simulink model "robot_TR4_joint"  (R2020a)
settings: Solver=ode15s  StartTime=0.0  StopTime=20.1113  RelTol=1e-3
undefined symbols (not defined in the file): dT_target, Fq_interp, Q_interp, Qp_interp, Qpp_interp, X, Y, Z
libraries: nesl_utility x25, sm_lib x18
settings Model: Creator=monti  LastModifiedBy=campr
settings DebuggingCC: SFMachineParentedDataDiag=error

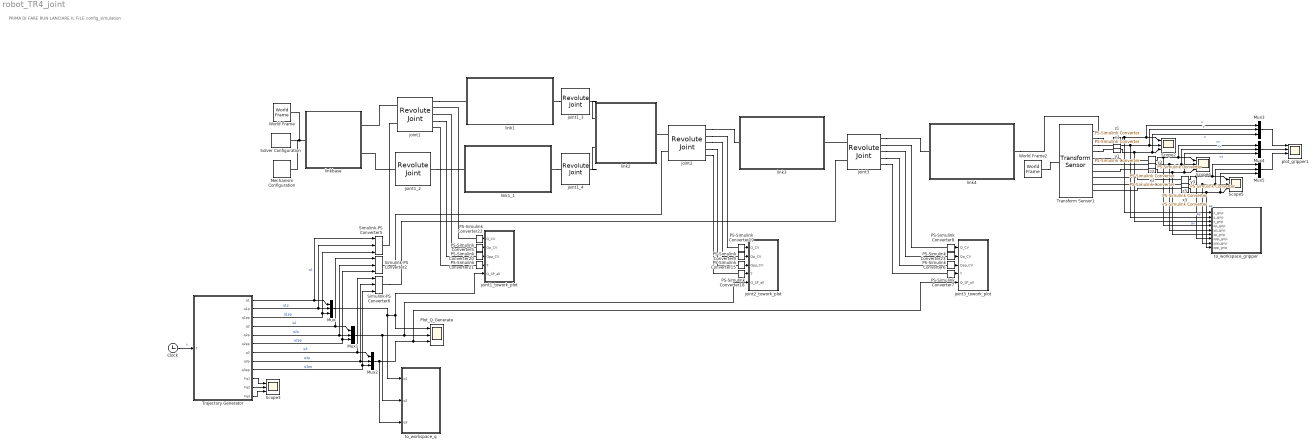
== system robot_TR4_joint ==
  note: PRIMA DI FARE RUN LANCIARE IL FILE config_simulation
  Clock : Clock
  Mechanism Configuration : sm_lib/Utilities/Mechanism Configuration  UniformGravity=Constant  GravityVector=[0 -9.80665 0]  GravityVectorUnits=m/s^2  GravityUnits=m/s^2  LinearizationDelta=0.001  JointModeTransitionNonlinearIterations=2
  Mux{,1..5} (6 alike) : Mux  Inputs=3
  PS-Simulink Converter15 : nesl_utility/PS-Simulink Converter  PhysicalDomain=network_engine_domain  SubClassName=ps_output  LeftPortType=input  RightPortType=output  PseudoPeriodic=off  Frequencies=[]  Unit=rad/s^2  AffineConversion=off
  PS-Simulink Converter18 : nesl_utility/PS-Simulink Converter  PhysicalDomain=network_engine_domain  SubClassName=ps_output  LeftPortType=input  RightPortType=output  PseudoPeriodic=off  Frequencies=[]  Unit=N*m  AffineConversion=off
  PS-Simulink Converter19 : nesl_utility/PS-Simulink Converter  PhysicalDomain=network_engine_domain  SubClassName=ps_output  LeftPortType=input  RightPortType=output  PseudoPeriodic=off  Frequencies=[]  Unit=rad  AffineConversion=off
  PS-Simulink Converter20 : nesl_utility/PS-Simulink Converter  PhysicalDomain=network_engine_domain  SubClassName=ps_output  LeftPortType=input  RightPortType=output  PseudoPeriodic=off  Frequencies=[]  Unit=rad/s^2  AffineConversion=off
  PS-Simulink Converter21 : nesl_utility/PS-Simulink Converter  PhysicalDomain=network_engine_domain  SubClassName=ps_output  LeftPortType=input  RightPortType=output  PseudoPeriodic=off  Frequencies=[]  Unit=N*m  AffineConversion=off
  PS-Simulink Converter22 : nesl_utility/PS-Simulink Converter  PhysicalDomain=network_engine_domain  SubClassName=ps_output  LeftPortType=input  RightPortType=output  PseudoPeriodic=off  Frequencies=[]  Unit=rad  AffineConversion=off
  PS-Simulink Converter23 : nesl_utility/PS-Simulink Converter  PhysicalDomain=network_engine_domain  SubClassName=ps_output  LeftPortType=input  RightPortType=output  PseudoPeriodic=off  Frequencies=[]  Unit=rad/s  AffineConversion=off
  PS-Simulink Converter5 : nesl_utility/PS-Simulink Converter  PhysicalDomain=network_engine_domain  SubClassName=ps_output  LeftPortType=input  RightPortType=output  PseudoPeriodic=off  Frequencies=[]  Unit=rad/s  AffineConversion=off
  PS-Simulink Converter6 : nesl_utility/PS-Simulink Converter  PhysicalDomain=network_engine_domain  SubClassName=ps_output  LeftPortType=input  RightPortType=output  PseudoPeriodic=off  Frequencies=[]  Unit=rad/s^2  AffineConversion=off
  PS-Simulink Converter7 : nesl_utility/PS-Simulink Converter  PhysicalDomain=network_engine_domain  SubClassName=ps_output  LeftPortType=input  RightPortType=output  PseudoPeriodic=off  Frequencies=[]  Unit=N*m  AffineConversion=off
  PS-Simulink Converter8 : nesl_utility/PS-Simulink Converter  PhysicalDomain=network_engine_domain  SubClassName=ps_output  LeftPortType=input  RightPortType=output  PseudoPeriodic=off  Frequencies=[]  Unit=rad  AffineConversion=off
  PS-Simulink Converter9 : nesl_utility/PS-Simulink Converter  PhysicalDomain=network_engine_domain  SubClassName=ps_output  LeftPortType=input  RightPortType=output  PseudoPeriodic=off  Frequencies=[]  Unit=rad/s  AffineConversion=off
  Plot_Q_Generate : Scope  NumInputPorts=3
  Scope{2..5} (4 alike) : Scope  NumInputPorts=3
  Simulink-PS Converter2 : nesl_utility/Simulink-PS Converter  PhysicalDomain=network_engine_domain  SubClassName=ps_input  LeftPortType=input  RightPortType=output  PseudoPeriodic=off  Frequencies=[]  NoiseDistribution=none  NoiseParameters=[]  Unit=rad  AffineConversion=off  FilteringAndDerivatives=provide  SimscapeFilterOrder=1  InputFilterTimeConstant=0.001  UdotUserProvided=2
  Simulink-PS Converter5 : nesl_utility/Simulink-PS Converter  PhysicalDomain=network_engine_domain  SubClassName=ps_input  LeftPortType=input  RightPortType=output  PseudoPeriodic=off  Frequencies=[]  NoiseDistribution=none  NoiseParameters=[]  Unit=rad  AffineConversion=off  FilteringAndDerivatives=provide  SimscapeFilterOrder=1  InputFilterTimeConstant=0.001  UdotUserProvided=2
  Simulink-PS Converter6 : nesl_utility/Simulink-PS Converter  PhysicalDomain=network_engine_domain  SubClassName=ps_input  LeftPortType=input  RightPortType=output  PseudoPeriodic=off  Frequencies=[]  NoiseDistribution=none  NoiseParameters=[]  Unit=rad  AffineConversion=off  FilteringAndDerivatives=provide  SimscapeFilterOrder=1  InputFilterTimeConstant=0.001  UdotUserProvided=2
  Solver Configuration : nesl_utility/Solver Configuration  PhysicalDomain=network_engine_domain  SubClassName=solver  LeftPortType=input  RightPortType=generic  Tones=[]  Harmonics=[]  SimulateNoise=off  Profile=off  UseLocalSampling=off  EnableSwitchedLinearOptims=on  FrequencyDomain=off  UseCCode=off  RelTol=0.001  AbsTol=1e-06  MinStep=1e-09  ToWorkspace=off  RevertToSquareIcSolve=off  NumHomotopyIterations=100  PhasorMode=off  PhasorModeNumHarmonics=1  DoDC=off  ResidualTolerance=1e-5  UseLocalSolver=off  LocalSolverChoice=NE_BACKWARD_EULER_ADVANCER  LocalSolverSampleTime=0.001  DoFixedCost=off  MaxNonlinIter=3  MaxModeIter=2  ComputeImpulses=off  ImpulseIterations=2  LinearAlgebra=Sparse  EquationFormulation=NE_TIME_EF  DelaysMemoryBudget=1024  AutomaticFiltering=on  FilteringTimeConstant=0.001  PartitionStorageMethod=AS_NEEDED  PartitionMemoryBudget=1024  PartitionMethod=FAST
  Trajectory Generator : MATLAB Function  TreatAsAtomicUnit=on
  Transform Sensor1 : sm_lib/Frames and Transforms/Transform Sensor  MeasurementFrame=World  SenseAngle=off  SenseAxis=off  SenseAngle1=off  SenseAngle2=off  SenseAngle3=off  SenseQ=off  SenseR=off  SenseOmegaX=off  SenseOmegaY=off  SenseOmegaZ=off  SenseOmega1=off  SenseOmega2=off  SenseOmega3=off  SenseQDot=off  SenseRDot=off  SenseAlphaX=off  SenseAlphaY=off  SenseAlphaZ=off  SenseAlpha1=off  SenseAlpha2=off  SenseAlpha3=off  SenseQDDot=off  SenseRDDot=off  SenseX=on  SenseY=on  SenseZ=on  SenseRad=off  SenseAzim=off  SenseDist=off  SenseInc=off  SenseXDot=on  SenseYDot=on  SenseZDot=on  SenseRadDot=off  SenseAzimDot=off  SenseDistDot=off  SenseIncDot=off  SenseXDDot=on  SenseYDDot=on  SenseZDDot=on  SenseRadDDot=off  SenseAzimDDot=off  SenseDistDDot=off  SenseIncDDot=off
  World Frame : sm_lib/Frames and Transforms/World Frame
  World Frame2 : sm_lib/Frames and Transforms/World Frame
  joint1 : sm_lib/Joints/Revolute Joint  JointMode=Normal  SenseConstraintForce=off  SenseConstraintForceX=off  SenseConstraintForceY=off  SenseConstraintForceZ=off  SenseConstraintTorque=off  SenseConstraintTorqueX=off  SenseConstraintTorqueY=off  SenseConstraintTorqueZ=off  SenseTotalForce=off  SenseTotalForceX=off  SenseTotalForceY=off  SenseTotalForceZ=off  SenseTotalTorque=off  SenseTotalTorqueX=off  SenseTotalTorqueY=off  SenseTotalTorqueZ=off  CompositeWrenchDir=FollowerOnBase  CompositeWrenchFrame=BaseFrame  EquilibriumPosition=0  EquilibriumPositionUnits=rad  SpringStiffness=0  SpringStiffnessUnits=N*m/deg  DampingCoefficient=0  DampingCoefficientUnits=N*m/(deg/s)  TorqueActuationMode=ComputedTorque  MotionActuationMode=InputMotion  SensePosition=on  SenseVelocity=on  SenseAcceleration=on  SenseTorqueForce=on  SenseLowerLimitTorqueForce=off  SenseUpperLimitTorqueForce=off  LowerLimitSpecify=on  LowerLimitBound=-1.5708  LowerLimitBoundUnits=rad  LowerLimitStiffness=0  LowerLimitStiffnessUnits=N*m/deg  LowerLimitDamping=0  LowerLimitDampingUnits=N*m/(deg/s)  LowerLimitTransitionRegionWidth=0.1  LowerLimitTransitionRegionWidthUnits=deg  UpperLimitSpecify=on  UpperLimitBound=1.5708  UpperLimitBoundUnits=rad  UpperLimitStiffness=0  UpperLimitStiffnessUnits=N*m/deg  UpperLimitDamping=0  UpperLimitDampingUnits=N*m/(deg/s)  UpperLimitTransitionRegionWidth=0.1  UpperLimitTransitionRegionWidthUnits=deg  PositionTargetSpecify=on  PositionTargetPriority=High  PositionTargetValue=0.5236  PositionTargetValueUnits=rad  VelocityTargetSpecify=off  VelocityTargetPriority=High  VelocityTargetValue=10  VelocityTargetValueUnits=deg/s
  joint1_2 : sm_lib/Joints/Revolute Joint  JointMode=Normal  SenseConstraintForce=off  SenseConstraintForceX=off  SenseConstraintForceY=off  SenseConstraintForceZ=off  SenseConstraintTorque=off  SenseConstraintTorqueX=off  SenseConstraintTorqueY=off  SenseConstraintTorqueZ=off  SenseTotalForce=off  SenseTotalForceX=off  SenseTotalForceY=off  SenseTotalForceZ=off  SenseTotalTorque=off  SenseTotalTorqueX=off  SenseTotalTorqueY=off  SenseTotalTorqueZ=off  CompositeWrenchDir=FollowerOnBase  CompositeWrenchFrame=BaseFrame  EquilibriumPosition=0  EquilibriumPositionUnits=deg  SpringStiffness=0  SpringStiffnessUnits=N*m/deg  DampingCoefficient=0  DampingCoefficientUnits=N*m/(deg/s)  TorqueActuationMode=NoTorque  MotionActuationMode=ComputedMotion  SensePosition=off  SenseVelocity=off  SenseAcceleration=off  SenseTorqueForce=off  SenseLowerLimitTorqueForce=off  SenseUpperLimitTorqueForce=off  LowerLimitSpecify=off  LowerLimitBound=-1.5708  LowerLimitBoundUnits=rad  LowerLimitStiffness=1e4  LowerLimitStiffnessUnits=N*m/deg  LowerLimitDamping=10  LowerLimitDampingUnits=N*m/(deg/s)  LowerLimitTransitionRegionWidth=0.1  LowerLimitTransitionRegionWidthUnits=deg  UpperLimitSpecify=off  UpperLimitBound=1.5708  UpperLimitBoundUnits=rad  UpperLimitStiffness=1e4  UpperLimitStiffnessUnits=N*m/deg  UpperLimitDamping=10  UpperLimitDampingUnits=N*m/(deg/s)  UpperLimitTransitionRegionWidth=0.1  UpperLimitTransitionRegionWidthUnits=deg  PositionTargetSpecify=on  PositionTargetPriority=High  PositionTargetValue=0.5236  PositionTargetValueUnits=rad  VelocityTargetSpecify=off  VelocityTargetPriority=High  VelocityTargetValue=0  VelocityTargetValueUnits=deg/s
  joint1_3 : sm_lib/Joints/Revolute Joint  JointMode=Normal  SenseConstraintForce=off  SenseConstraintForceX=off  SenseConstraintForceY=off  SenseConstraintForceZ=off  SenseConstraintTorque=off  SenseConstraintTorqueX=off  SenseConstraintTorqueY=off  SenseConstraintTorqueZ=off  SenseTotalForce=off  SenseTotalForceX=off  SenseTotalForceY=off  SenseTotalForceZ=off  SenseTotalTorque=off  SenseTotalTorqueX=off  SenseTotalTorqueY=off  SenseTotalTorqueZ=off  CompositeWrenchDir=FollowerOnBase  CompositeWrenchFrame=BaseFrame  EquilibriumPosition=0  EquilibriumPositionUnits=deg  SpringStiffness=0  SpringStiffnessUnits=N*m/deg  DampingCoefficient=0  DampingCoefficientUnits=N*m/(deg/s)  TorqueActuationMode=NoTorque  MotionActuationMode=ComputedMotion  SensePosition=off  SenseVelocity=off  SenseAcceleration=off  SenseTorqueForce=off  SenseLowerLimitTorqueForce=off  SenseUpperLimitTorqueForce=off  LowerLimitSpecify=off  LowerLimitBound=-90  LowerLimitBoundUnits=deg  LowerLimitStiffness=1e4  LowerLimitStiffnessUnits=N*m/deg  LowerLimitDamping=10  LowerLimitDampingUnits=N*m/(deg/s)  LowerLimitTransitionRegionWidth=0.1  LowerLimitTransitionRegionWidthUnits=deg  UpperLimitSpecify=off  UpperLimitBound=90  UpperLimitBoundUnits=deg  UpperLimitStiffness=1e4  UpperLimitStiffnessUnits=N*m/deg  UpperLimitDamping=10  UpperLimitDampingUnits=N*m/(deg/s)  UpperLimitTransitionRegionWidth=0.1  UpperLimitTransitionRegionWidthUnits=deg  PositionTargetSpecify=off  PositionTargetPriority=High  PositionTargetValue=0  PositionTargetValueUnits=deg  VelocityTargetSpecify=off  VelocityTargetPriority=High  VelocityTargetValue=0  VelocityTargetValueUnits=deg/s
  joint1_4 : sm_lib/Joints/Revolute Joint  JointMode=Normal  SenseConstraintForce=off  SenseConstraintForceX=off  SenseConstraintForceY=off  SenseConstraintForceZ=off  SenseConstraintTorque=off  SenseConstraintTorqueX=off  SenseConstraintTorqueY=off  SenseConstraintTorqueZ=off  SenseTotalForce=off  SenseTotalForceX=off  SenseTotalForceY=off  SenseTotalForceZ=off  SenseTotalTorque=off  SenseTotalTorqueX=off  SenseTotalTorqueY=off  SenseTotalTorqueZ=off  CompositeWrenchDir=FollowerOnBase  CompositeWrenchFrame=BaseFrame  EquilibriumPosition=0  EquilibriumPositionUnits=deg  SpringStiffness=0  SpringStiffnessUnits=N*m/deg  DampingCoefficient=0  DampingCoefficientUnits=N*m/(deg/s)  TorqueActuationMode=NoTorque  MotionActuationMode=ComputedMotion  SensePosition=off  SenseVelocity=off  SenseAcceleration=off  SenseTorqueForce=off  SenseLowerLimitTorqueForce=off  SenseUpperLimitTorqueForce=off  LowerLimitSpecify=off  LowerLimitBound=-90  LowerLimitBoundUnits=deg  LowerLimitStiffness=1e4  LowerLimitStiffnessUnits=N*m/deg  LowerLimitDamping=10  LowerLimitDampingUnits=N*m/(deg/s)  LowerLimitTransitionRegionWidth=0.1  LowerLimitTransitionRegionWidthUnits=deg  UpperLimitSpecify=off  UpperLimitBound=90  UpperLimitBoundUnits=deg  UpperLimitStiffness=1e4  UpperLimitStiffnessUnits=N*m/deg  UpperLimitDamping=10  UpperLimitDampingUnits=N*m/(deg/s)  UpperLimitTransitionRegionWidth=0.1  UpperLimitTransitionRegionWidthUnits=deg  PositionTargetSpecify=off  PositionTargetPriority=High  PositionTargetValue=0  PositionTargetValueUnits=deg  VelocityTargetSpecify=off  VelocityTargetPriority=High  VelocityTargetValue=0  VelocityTargetValueUnits=deg/s
  joint1_towork_plot : Subsystem
  joint2 : sm_lib/Joints/Revolute Joint  JointMode=Normal  SenseConstraintForce=off  SenseConstraintForceX=off  SenseConstraintForceY=off  SenseConstraintForceZ=off  SenseConstraintTorque=off  SenseConstraintTorqueX=off  SenseConstraintTorqueY=off  SenseConstraintTorqueZ=off  SenseTotalForce=off  SenseTotalForceX=off  SenseTotalForceY=off  SenseTotalForceZ=off  SenseTotalTorque=off  SenseTotalTorqueX=off  SenseTotalTorqueY=off  SenseTotalTorqueZ=off  CompositeWrenchDir=FollowerOnBase  CompositeWrenchFrame=BaseFrame  EquilibriumPosition=0  EquilibriumPositionUnits=deg  SpringStiffness=0  SpringStiffnessUnits=N*m/deg  DampingCoefficient=0  DampingCoefficientUnits=N*m/(deg/s)  TorqueActuationMode=ComputedTorque  MotionActuationMode=InputMotion  SensePosition=on  SenseVelocity=on  SenseAcceleration=on  SenseTorqueForce=on  SenseLowerLimitTorqueForce=off  SenseUpperLimitTorqueForce=off  LowerLimitSpecify=on  LowerLimitBound=-1.9199  LowerLimitBoundUnits=rad  LowerLimitStiffness=0  LowerLimitStiffnessUnits=N*m/deg  LowerLimitDamping=0  LowerLimitDampingUnits=N*m/(deg/s)  LowerLimitTransitionRegionWidth=0.1  LowerLimitTransitionRegionWidthUnits=deg  UpperLimitSpecify=on  UpperLimitBound=1.9199  UpperLimitBoundUnits=rad  UpperLimitStiffness=0  UpperLimitStiffnessUnits=N*m/deg  UpperLimitDamping=0  UpperLimitDampingUnits=N*m/(deg/s)  UpperLimitTransitionRegionWidth=0.1  UpperLimitTransitionRegionWidthUnits=deg  PositionTargetSpecify=on  PositionTargetPriority=High  PositionTargetValue=0.5236  PositionTargetValueUnits=rad  VelocityTargetSpecify=off  VelocityTargetPriority=High  VelocityTargetValue=0  VelocityTargetValueUnits=deg/s
  joint2_towork_plot : Subsystem
  joint3 : sm_lib/Joints/Revolute Joint  JointMode=Normal  SenseConstraintForce=off  SenseConstraintForceX=off  SenseConstraintForceY=off  SenseConstraintForceZ=off  SenseConstraintTorque=off  SenseConstraintTorqueX=off  SenseConstraintTorqueY=off  SenseConstraintTorqueZ=off  SenseTotalForce=off  SenseTotalForceX=off  SenseTotalForceY=off  SenseTotalForceZ=off  SenseTotalTorque=off  SenseTotalTorqueX=off  SenseTotalTorqueY=off  SenseTotalTorqueZ=off  CompositeWrenchDir=FollowerOnBase  CompositeWrenchFrame=BaseFrame  EquilibriumPosition=0  EquilibriumPositionUnits=deg  SpringStiffness=0  SpringStiffnessUnits=N*m/deg  DampingCoefficient=0  DampingCoefficientUnits=N*m/(deg/s)  TorqueActuationMode=ComputedTorque  MotionActuationMode=InputMotion  SensePosition=on  SenseVelocity=on  SenseAcceleration=on  SenseTorqueForce=on  SenseLowerLimitTorqueForce=off  SenseUpperLimitTorqueForce=off  LowerLimitSpecify=on  LowerLimitBound=-2.2689  LowerLimitBoundUnits=rad  LowerLimitStiffness=0  LowerLimitStiffnessUnits=N*m/deg  LowerLimitDamping=0  LowerLimitDampingUnits=N*m/(deg/s)  LowerLimitTransitionRegionWidth=0.1  LowerLimitTransitionRegionWidthUnits=deg  UpperLimitSpecify=on  UpperLimitBound=2.2689  UpperLimitBoundUnits=rad  UpperLimitStiffness=0  UpperLimitStiffnessUnits=N*m/deg  UpperLimitDamping=0  UpperLimitDampingUnits=N*m/(deg/s)  UpperLimitTransitionRegionWidth=0.1  UpperLimitTransitionRegionWidthUnits=deg  PositionTargetSpecify=on  PositionTargetPriority=High  PositionTargetValue=0.5236  PositionTargetValueUnits=rad  VelocityTargetSpecify=off  VelocityTargetPriority=High  VelocityTargetValue=0  VelocityTargetValueUnits=deg/s
  joint3_towork_plot : Subsystem
  link1 : Subsystem
      mask Display: image('$imagefile'); % Use "Edit Image" on toolstrip to change.
  link1_1 : Subsystem
      mask Display: image('$imagefile'); % Use "Edit Image" on toolstrip to change.
  link2 : Subsystem
      mask Display: image('$imagefile'); % Use "Edit Image" on toolstrip to change.
  link3 : Subsystem
      mask Display: image('$imagefile'); % Use "Edit Image" on toolstrip to change.
  link4 : Subsystem
      mask Display: image('$imagefile'); % Use "Edit Image" on toolstrip to change.
  linkbase : Subsystem  mask{offset=15}
      mask Display: image('$imagefile'); % Use "Edit Image" on toolstrip to change.
  plot_gripper1 : Scope  NumInputPorts=4
  to_workspace_gripper : Subsystem
  to_workspace_q : Subsystem
  x1 : nesl_utility/PS-Simulink Converter  PhysicalDomain=network_engine_domain  SubClassName=ps_output  LeftPortType=input  RightPortType=output  PseudoPeriodic=off  Frequencies=[]  Unit=m  AffineConversion=off
  x2 : nesl_utility/PS-Simulink Converter  PhysicalDomain=network_engine_domain  SubClassName=ps_output  LeftPortType=input  RightPortType=output  PseudoPeriodic=off  Frequencies=[]  Unit=m/s  AffineConversion=off
  x3 : nesl_utility/PS-Simulink Converter  PhysicalDomain=network_engine_domain  SubClassName=ps_output  LeftPortType=input  RightPortType=output  PseudoPeriodic=off  Frequencies=[]  Unit=m/s^2  AffineConversion=off
  y1 : nesl_utility/PS-Simulink Converter  PhysicalDomain=network_engine_domain  SubClassName=ps_output  LeftPortType=input  RightPortType=output  PseudoPeriodic=off  Frequencies=[]  Unit=m  AffineConversion=off
  y2 : nesl_utility/PS-Simulink Converter  PhysicalDomain=network_engine_domain  SubClassName=ps_output  LeftPortType=input  RightPortType=output  PseudoPeriodic=off  Frequencies=[]  Unit=m/s  AffineConversion=off
  y3 : nesl_utility/PS-Simulink Converter  PhysicalDomain=network_engine_domain  SubClassName=ps_output  LeftPortType=input  RightPortType=output  PseudoPeriodic=off  Frequencies=[]  Unit=m/s^2  AffineConversion=off
  z1 : nesl_utility/PS-Simulink Converter  PhysicalDomain=network_engine_domain  SubClassName=ps_output  LeftPortType=input  RightPortType=output  PseudoPeriodic=off  Frequencies=[]  Unit=m  AffineConversion=off
  z2 : nesl_utility/PS-Simulink Converter  PhysicalDomain=network_engine_domain  SubClassName=ps_output  LeftPortType=input  RightPortType=output  PseudoPeriodic=off  Frequencies=[]  Unit=m/s  AffineConversion=off
  z3 : nesl_utility/PS-Simulink Converter  PhysicalDomain=network_engine_domain  SubClassName=ps_output  LeftPortType=input  RightPortType=output  PseudoPeriodic=off  Frequencies=[]  Unit=m/s^2  AffineConversion=off
  wires:
  Clock/1 -> Trajectory Generator/1(t)  "t"
  x1/1 -> to_workspace_gripper/3(z_grip), Mux3/3, Scope2/3  "z"
  Trajectory Generator/12(Fq3) -> Scope3/3
  Mux3/1 -> plot_gripper1/1
  Trajectory Generator/10(Fq1) -> Scope3/1
  PS-Simulink Converter22/1 -> joint1_towork_plot/1(Q_CV)
  Mux5/1 -> plot_gripper1/3
  PS-Simulink Converter9/1 -> joint2_towork_plot/2(Qp_CV)
  z3/1 -> to_workspace_gripper/7(xpp_grip), Mux5/1, Scope5/1  "ax"
  Mux1/1 -> Plot_Q_Generate/2, joint2_towork_plot/5(Q_SP_all), to_workspace_q/2(q2)
  PS-Simulink Converter15/1 -> joint2_towork_plot/3(Qpp_CV)
  Trajectory Generator/11(Fq2) -> Scope3/2
  Trajectory Generator/1(q1) -> Mux/1, Simulink-PS Converter5/1  "q1"
  PS-Simulink Converter18/1 -> joint2_towork_plot/4(T)
  y2/1 -> to_workspace_gripper/5(yp_grip), Mux4/2, Scope4/2  "vy"
  PS-Simulink Converter19/1 -> joint2_towork_plot/1(Q_CV)
  z1/1 -> to_workspace_gripper/1(x_grip), Mux3/1, Scope2/1  "x"
  PS-Simulink Converter7/1 -> joint3_towork_plot/4(T)
  PS-Simulink Converter20/1 -> joint1_towork_plot/3(Qpp_CV)
  Trajectory Generator/8(q3p) -> Simulink-PS Converter6/2, Mux2/2  "q3p"
  Mux/1 -> to_workspace_q/1(q1), joint1_towork_plot/5(Q_SP_all), Plot_Q_Generate/1
  PS-Simulink Converter8/1 -> joint3_towork_plot/1(Q_CV)
  PS-Simulink Converter6/1 -> joint3_towork_plot/3(Qpp_CV)
  PS-Simulink Converter23/1 -> joint3_towork_plot/2(Qp_CV)
  x2/1 -> to_workspace_gripper/6(zp_grip), Mux4/3, Scope4/3  "vz"
  Mux2/1 -> Plot_Q_Generate/3, joint3_towork_plot/5(Q_SP_all), to_workspace_q/3(q3)
  Trajectory Generator/5(q2p) -> Simulink-PS Converter2/2, Mux1/2  "q2p"
  Trajectory Generator/9(q3pp) -> Simulink-PS Converter6/3, Mux2/3  "q3pp"
  PS-Simulink Converter21/1 -> joint1_towork_plot/4(T)
  x3/1 -> Mux5/3, Scope5/3, to_workspace_gripper/9(zpp_grip)  "az"
  z2/1 -> Mux4/1, Scope4/1, to_workspace_gripper/4(xp_grip)  "vx"
  Mux4/1 -> plot_gripper1/2
  Trajectory Generator/4(q2) -> Mux1/1, Simulink-PS Converter2/1  "q2"
  y1/1 -> to_workspace_gripper/2(y_grip), Mux3/2, Scope2/2  "y"
  Trajectory Generator/2(q1p) -> Mux/2, Simulink-PS Converter5/2  "q1p"
  PS-Simulink Converter5/1 -> joint1_towork_plot/2(Qp_CV)
  y3/1 -> Mux5/2, Scope5/2, to_workspace_gripper/8(ypp_grip)  "ay"
  Trajectory Generator/3(q1pp) -> Mux/3, Simulink-PS Converter5/3  "q1pp"
  Trajectory Generator/7(q3) -> Simulink-PS Converter6/1, Mux2/1  "q3"
  Trajectory Generator/6(q2pp) -> Simulink-PS Converter2/3, Mux1/3  "q2pp"
  connections:
  linkbase/LConn1 -- Mechanism Configuration/RConn1 -- World Frame/RConn1 -- Solver Configuration/RConn1
  Transform Sensor1/RConn3 -- y1/LConn1
  Transform Sensor1/RConn2 -- z1/LConn1
  PS-Simulink Converter21/LConn1 -- joint1/RConn5
  y2/LConn1 -- Transform Sensor1/RConn6
  joint2/RConn3 -- PS-Simulink Converter9/LConn1
  joint3/RConn5 -- PS-Simulink Converter7/LConn1
  joint3/RConn3 -- PS-Simulink Converter23/LConn1
  PS-Simulink Converter22/LConn1 -- joint1/RConn2
  PS-Simulink Converter5/LConn1 -- joint1/RConn3
  joint3/RConn4 -- PS-Simulink Converter6/LConn1
  joint1_2/LConn1 -- linkbase/RConn2
  joint1/LConn1 -- linkbase/RConn1
  joint2/RConn5 -- PS-Simulink Converter18/LConn1
  joint3/RConn2 -- PS-Simulink Converter8/LConn1
  joint1/RConn1 -- link1/LConn1
  x2/LConn1 -- Transform Sensor1/RConn7
  joint1/RConn4 -- PS-Simulink Converter20/LConn1
  joint2/RConn4 -- PS-Simulink Converter15/LConn1
  y3/LConn1 -- Transform Sensor1/RConn9
  joint1_4/RConn1 -- link2/LConn2
  joint1_3/RConn1 -- link2/LConn1
  joint3/LConn1 -- link3/RConn1
  x3/LConn1 -- Transform Sensor1/RConn10
  link4/RConn1 -- Transform Sensor1/RConn1
  z2/LConn1 -- Transform Sensor1/RConn5
  Transform Sensor1/RConn4 -- x1/LConn1
  World Frame2/RConn1 -- Transform Sensor1/LConn1
  joint2/LConn1 -- link2/RConn1
  link1/RConn1 -- joint1_3/LConn1
  joint3/RConn1 -- link4/LConn1
  joint1_2/RConn1 -- link1_1/LConn1
  joint2/RConn1 -- link3/LConn1
  link1_1/RConn1 -- joint1_4/LConn1
  z3/LConn1 -- Transform Sensor1/RConn8
  joint2/RConn2 -- PS-Simulink Converter19/LConn1
  Simulink-PS Converter5/RConn1 -- joint1/LConn2
  Simulink-PS Converter2/RConn1 -- joint2/LConn2
  Simulink-PS Converter6/RConn1 -- joint3/LConn2

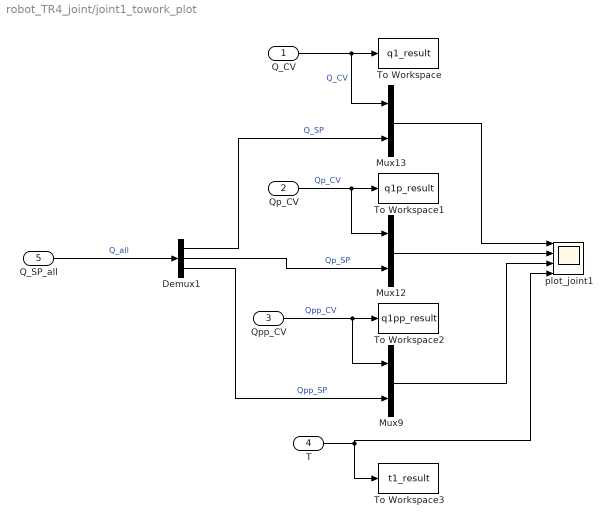
== system robot_TR4_joint/joint1_towork_plot ==
  Q_CV : Inport
  Qp_CV : Inport  Port=2
  Qpp_CV : Inport  Port=3
  T : Inport  Port=4
  Q_SP_all : Inport  Port=5
  Demux1 : Demux  Outputs=3
  Mux12 : Mux  Inputs=2
  Mux13 : Mux  Inputs=2
  Mux9 : Mux  Inputs=2
  To Workspace : ToWorkspace  VariableName=q1_result  SaveFormat=Timeseries  SampleTime=-1
  To Workspace1 : ToWorkspace  VariableName=q1p_result  SaveFormat=Timeseries  SampleTime=-1
  To Workspace2 : ToWorkspace  VariableName=q1pp_result  SaveFormat=Timeseries  SampleTime=-1
  To Workspace3 : ToWorkspace  VariableName=t1_result  SaveFormat=Timeseries  SampleTime=-1
  plot_joint1 : Scope  NumInputPorts=4
  wires:
  Demux1/1 -> Mux13/2  "Q_SP"
  Demux1/2 -> Mux12/2  "Qp_SP"
  Qpp_CV/1 -> Mux9/1, To Workspace2/1  "Qpp_CV"
  Qp_CV/1 -> Mux12/1, To Workspace1/1  "Qp_CV"
  Q_CV/1 -> Mux13/1, To Workspace/1  "Q_CV"
  T/1 -> plot_joint1/4, To Workspace3/1
  Demux1/3 -> Mux9/2  "Qpp_SP"
  Q_SP_all/1 -> Demux1/1  "Q_all"
  Mux13/1 -> plot_joint1/1
  Mux12/1 -> plot_joint1/2
  Mux9/1 -> plot_joint1/3

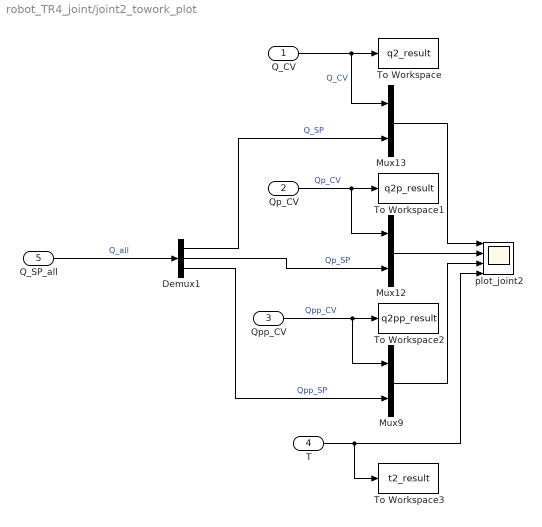
== system robot_TR4_joint/joint2_towork_plot ==
  Q_CV : Inport
  Qp_CV : Inport  Port=2
  Qpp_CV : Inport  Port=3
  T : Inport  Port=4
  Q_SP_all : Inport  Port=5
  Demux1 : Demux  Outputs=3
  Mux12 : Mux  Inputs=2
  Mux13 : Mux  Inputs=2
  Mux9 : Mux  Inputs=2
  To Workspace : ToWorkspace  VariableName=q2_result  SaveFormat=Timeseries  SampleTime=-1
  To Workspace1 : ToWorkspace  VariableName=q2p_result  SaveFormat=Timeseries  SampleTime=-1
  To Workspace2 : ToWorkspace  VariableName=q2pp_result  SaveFormat=Timeseries  SampleTime=-1
  To Workspace3 : ToWorkspace  VariableName=t2_result  SaveFormat=Timeseries  SampleTime=-1
  plot_joint2 : Scope  NumInputPorts=4
  wires:
  Mux9/1 -> plot_joint2/3
  Demux1/1 -> Mux13/2  "Q_SP"
  Mux13/1 -> plot_joint2/1
  Mux12/1 -> plot_joint2/2
  Demux1/2 -> Mux12/2  "Qp_SP"
  Qpp_CV/1 -> Mux9/1, To Workspace2/1  "Qpp_CV"
  Qp_CV/1 -> Mux12/1, To Workspace1/1  "Qp_CV"
  Q_CV/1 -> Mux13/1, To Workspace/1  "Q_CV"
  T/1 -> To Workspace3/1, plot_joint2/4
  Demux1/3 -> Mux9/2  "Qpp_SP"
  Q_SP_all/1 -> Demux1/1  "Q_all"

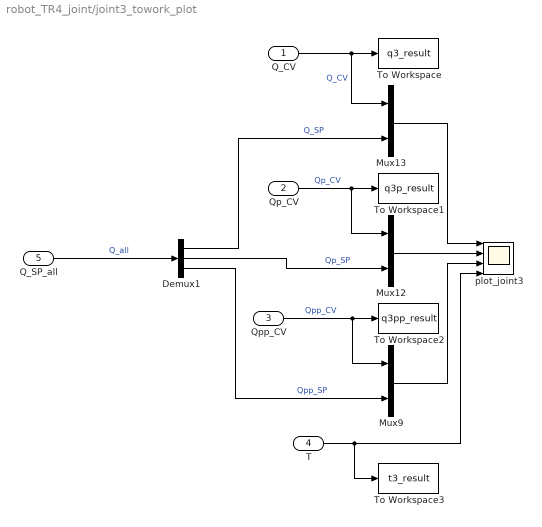
== system robot_TR4_joint/joint3_towork_plot ==
  Q_CV : Inport
  Qp_CV : Inport  Port=2
  Qpp_CV : Inport  Port=3
  T : Inport  Port=4
  Q_SP_all : Inport  Port=5
  Demux1 : Demux  Outputs=3
  Mux12 : Mux  Inputs=2
  Mux13 : Mux  Inputs=2
  Mux9 : Mux  Inputs=2
  To Workspace : ToWorkspace  VariableName=q3_result  SaveFormat=Timeseries  SampleTime=-1
  To Workspace1 : ToWorkspace  VariableName=q3p_result  SaveFormat=Timeseries  SampleTime=-1
  To Workspace2 : ToWorkspace  VariableName=q3pp_result  SaveFormat=Timeseries  SampleTime=-1
  To Workspace3 : ToWorkspace  VariableName=t3_result  SaveFormat=Timeseries  SampleTime=-1
  plot_joint3 : Scope  NumInputPorts=4
  wires:
  Mux9/1 -> plot_joint3/3
  Demux1/1 -> Mux13/2  "Q_SP"
  Mux13/1 -> plot_joint3/1
  Mux12/1 -> plot_joint3/2
  Demux1/2 -> Mux12/2  "Qp_SP"
  Qpp_CV/1 -> Mux9/1, To Workspace2/1  "Qpp_CV"
  Qp_CV/1 -> Mux12/1, To Workspace1/1  "Qp_CV"
  Q_CV/1 -> Mux13/1, To Workspace/1  "Q_CV"
  T/1 -> To Workspace3/1, plot_joint3/4
  Demux1/3 -> Mux9/2  "Qpp_SP"
  Q_SP_all/1 -> Demux1/1  "Q_all"

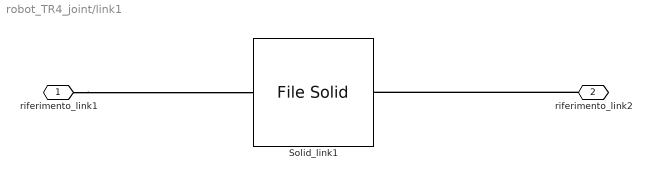
== system robot_TR4_joint/link1 ==
  Solid_link1 : sm_lib/Body Elements/File Solid  ExtGeomFileName=D:\repository\Servo_System_progetto\Solidworks\step\TR4link1.STEP  UnitType=FromFile  ExtGeomFileUnits=m  StepReaderType=HEX  ExportConvexHullGeometry=off  InertiaType=CalculateFromGeometry  Mass=2.64  MassUnits=g  CenterOfMass=[0 0 0]  CenterOfMassUnits=m  MomentsOfInertia=[1 1 1]  MomentsOfInertiaUnits=kg*m^2  ProductsOfInertia=[0 0 0]  ProductsOfInertiaUnits=kg*m^2  BasedOnType=Mass  Density=1  DensityUnits=kg/m^3  DoExposeReferenceFrame=off  SerializedFrames=<Frames><Frame><Id>Frame1</Id><Value><Name>BR1</Name><Origin><Source>GeometricFeature</Source><FeatureName>planar surface 5</FeatureName></Origin><PrimaryAxis><DefinedDirection>+Z</DefinedDirection><Source>ReferenceFrame</Source><SourceDirection>+Y</SourceDirection><FeatureName></FeatureName></PrimaryAxis><SecondaryAxis><DefinedDirection>+X</DefinedDirection><Source>ReferenceFrame</Source><SourceDirection>+X</SourceDirection><FeatureName></FeatureName></SecondaryAxis></Value></Frame><Frame><Id>Frame2</Id><Value><Name>RL1</Name><Origin><Source>GeometricFeature</Source><FeatureName>planar surface 7</FeatureName></Origin><PrimaryAxis><DefinedDirection>+Z</DefinedDirection><Source>GeometricFeature</Source><SourceDirection>+Z</SourceDirection><FeatureName>segment 10</FeatureName></PrimaryAxis><SecondaryAxis><DefinedDirection>+X</DefinedDirection><Source>ReferenceFrame</Source><SourceDirection>+X</SourceDirection><FeatureName></FeatureName></SecondaryAxis></Value></Frame></Frames>  GraphicType=FromGeometry  MarkerShape=Sphere  MarkerSize=10  GraphicVisPropType=SimpleVisualProperties  GraphicDiffuseColor=[0.5 0.5 0.5]  GraphicSpecularColor=[0.5 0.5 0.5 1.0]  GraphicAmbientColor=[0.15 0.15 0.15 1.0]  GraphicEmissiveColor=[0.0 0.0 0.0 1.0]  GraphicShininess=75  GraphicOpacity=1.0
  riferimento_link1 : PMIOPort  Side=Left
  riferimento_link2 : PMIOPort  Port=2  Side=Right
  connections:
  riferimento_link1/RConn1 -- Solid_link1/LConn1
  riferimento_link2/RConn1 -- Solid_link1/RConn1

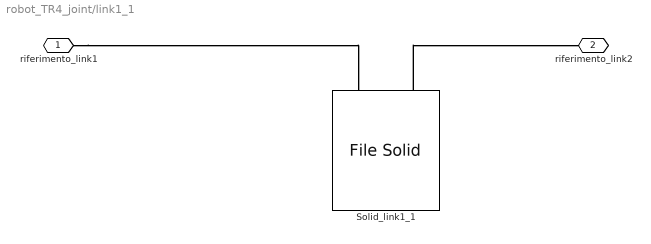
== system robot_TR4_joint/link1_1 ==
  Solid_link1_1 : sm_lib/Body Elements/File Solid  ExtGeomFileName=D:\repository\Servo_System_progetto\Solidworks\step\TR4link1.STEP  UnitType=FromFile  ExtGeomFileUnits=m  StepReaderType=HEX  ExportConvexHullGeometry=off  InertiaType=CalculateFromGeometry  Mass=2.64  MassUnits=g  CenterOfMass=[0 0 0]  CenterOfMassUnits=m  MomentsOfInertia=[1 1 1]  MomentsOfInertiaUnits=kg*m^2  ProductsOfInertia=[0 0 0]  ProductsOfInertiaUnits=kg*m^2  BasedOnType=Mass  Density=1  DensityUnits=kg/m^3  DoExposeReferenceFrame=on  SerializedFrames=<Frames><Frame><Id>Frame1</Id><Value><Name>BR1</Name><Origin><Source>GeometricFeature</Source><FeatureName>planar surface 5</FeatureName></Origin><PrimaryAxis><DefinedDirection>+Z</DefinedDirection><Source>GeometricFeature</Source><SourceDirection>+Z</SourceDirection><FeatureName>segment 13</FeatureName></PrimaryAxis><SecondaryAxis><DefinedDirection>+X</DefinedDirection><Source>ReferenceFrame</Source><SourceDirection>+X</SourceDirection><FeatureName></FeatureName></SecondaryAxis></Value></Frame><Frame><Id>Frame2</Id><Value><Name>RL1</Name><Origin><Source>GeometricFeature</Source><FeatureName>planar surface 7</FeatureName></Origin><PrimaryAxis><DefinedDirection>+Z</DefinedDirection><Source>GeometricFeature</Source><SourceDirection>+Z</SourceDirection><FeatureName>segment 10</FeatureName></PrimaryAxis><SecondaryAxis><DefinedDirection>+X</DefinedDirection><Source>ReferenceFrame</Source><SourceDirection>+X</SourceDirection><FeatureName></FeatureName></SecondaryAxis></Value></Frame></Frames>  GraphicType=FromGeometry  MarkerShape=Sphere  MarkerSize=10  GraphicVisPropType=SimpleVisualProperties  GraphicDiffuseColor=[0.5 0.5 0.5]  GraphicSpecularColor=[0.5 0.5 0.5 1.0]  GraphicAmbientColor=[0.15 0.15 0.15 1.0]  GraphicEmissiveColor=[0.0 0.0 0.0 1.0]  GraphicShininess=75  GraphicOpacity=1.0
  riferimento_link1 : PMIOPort  Side=Left
  riferimento_link2 : PMIOPort  Port=2  Side=Right
  connections:
  riferimento_link1/RConn1 -- Solid_link1_1/LConn1
  Solid_link1_1/LConn2 -- riferimento_link2/RConn1

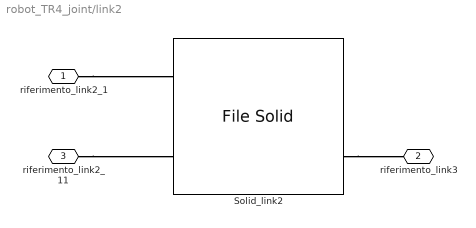
== system robot_TR4_joint/link2 ==
  Solid_link2 : sm_lib/Body Elements/File Solid  ExtGeomFileName=D:\repository\Servo_System_progetto\Solidworks\step\TR4link2.STEP  UnitType=FromFile  ExtGeomFileUnits=m  StepReaderType=HEX  ExportConvexHullGeometry=off  InertiaType=CalculateFromGeometry  Mass=4.12  MassUnits=g  CenterOfMass=[0 0 0]  CenterOfMassUnits=m  MomentsOfInertia=[1 1 1]  MomentsOfInertiaUnits=kg*m^2  ProductsOfInertia=[0 0 0]  ProductsOfInertiaUnits=kg*m^2  BasedOnType=Mass  Density=1  DensityUnits=kg/m^3  DoExposeReferenceFrame=on  SerializedFrames=<Frames><Frame><Id>Frame1</Id><Value><Name>R_L1</Name><Origin><Source>GeometricFeature</Source><FeatureName>circular curve 15</FeatureName></Origin><PrimaryAxis><DefinedDirection>+Z</DefinedDirection><Source>GeometricFeature</Source><SourceDirection>+Z</SourceDirection><FeatureName>segment 28</FeatureName></PrimaryAxis><SecondaryAxis><DefinedDirection>+X</DefinedDirection><Source>ReferenceFrame</Source><SourceDirection>+X</SourceDirection><FeatureName></FeatureName></SecondaryAxis></Value></Frame><Frame><Id>Frame2</Id><Value><Name>R_L2</Name><Origin><Source>GeometricFeature</Source><FeatureName>circular curve 26</FeatureName></Origin><PrimaryAxis><DefinedDirection>+Z</DefinedDirection><Source>GeometricFeature</Source><SourceDirection>+Z</SourceDirection><FeatureName>circular curve 26</FeatureName></PrimaryAxis><SecondaryAxis><DefinedDirection>+X</DefinedDirection><Source>ReferenceFrame</Source><SourceDirection>+X</SourceDirection><FeatureName></FeatureName></SecondaryAxis></Value></Frame><Frame><Id>Frame3</Id><Value><Name>R_23</Name><Origin><Source>GeometricFeature</Source><FeatureName>circular curve 31</FeatureName></Origin><PrimaryAxis><DefinedDirection>+Z</DefinedDirection><Source>GeometricFeature</Source><SourceDirection>+Z</SourceDirection><FeatureName>segment 37</FeatureName></PrimaryAxis><SecondaryAxis><DefinedDirection>+X</DefinedDirection><Source>ReferenceFrame</Source><SourceDirection>+X</SourceDirection><FeatureName></FeatureName></SecondaryAxis></Value></Frame></Frames>  GraphicType=FromGeometry  MarkerShape=Sphere  MarkerSize=10  GraphicVisPropType=SimpleVisualProperties  GraphicDiffuseColor=[0.5 0.5 0.5]  GraphicSpecularColor=[0.5 0.5 0.5 1.0]  GraphicAmbientColor=[0.15 0.15 0.15 1.0]  GraphicEmissiveColor=[0.0 0.0 0.0 1.0]  GraphicShininess=75  GraphicOpacity=1.0
  riferimento_link2_1 : PMIOPort  Side=Left
  riferimento_link3 : PMIOPort  Port=2  Side=Right
  riferimento_link2_11 : PMIOPort  Port=3  Side=Left
  connections:
  riferimento_link2_1/RConn1 -- Solid_link2/LConn1
  riferimento_link2_11/RConn1 -- Solid_link2/LConn2
  Solid_link2/RConn2 -- riferimento_link3/RConn1

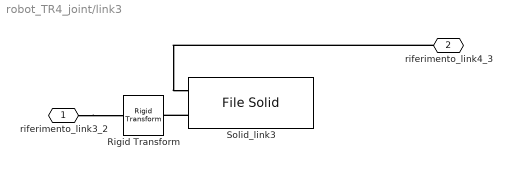
== system robot_TR4_joint/link3 ==
  Rigid Transform : sm_lib/Frames and Transforms/Rigid Transform  TranslationMethod=Cartesian  TranslationStandardOffset=0  TranslationLengthUnit=mm  TranslationStandardAxis=+Z  TranslationCartesianOffset=[0 0 -1]  TranslationROffset=0  TranslationROffsetUnits=m  TranslationZOffset=0  TranslationZOffsetUnits=m  TranslationThetaOffset=0  TranslationThetaOffsetUnits=deg  RotationMethod=StandardAxis  RotationAngleUnits=deg  RotationStandardAxis=+Z  RotationAngle=90  RotationArbitraryAxis=[0 0 1]  FollAlignAxisA=+X  BaseAlignAxisA=+Y  FollAlignAxisB=+Y  BaseAlignAxisB=+Z  RotationSequenceAxes=FollowerAxes  RotationSequence=XYX  RotationSequenceAngles=[0 0 0]  RotationSequenceAnglesUnits=deg  RotationMatrix=[1 0 0; 0 1 0; 0 0 1]
  Solid_link3 : sm_lib/Body Elements/File Solid  ExtGeomFileName=D:\repository\Servo_System_progetto\Solidworks\step\TR4link3.STEP  UnitType=FromFile  ExtGeomFileUnits=m  StepReaderType=HEX  ExportConvexHullGeometry=off  InertiaType=CalculateFromGeometry  Mass=4.05  MassUnits=g  CenterOfMass=[0 0 0]  CenterOfMassUnits=m  MomentsOfInertia=[1 1 1]  MomentsOfInertiaUnits=kg*m^2  ProductsOfInertia=[0 0 0]  ProductsOfInertiaUnits=kg*m^2  BasedOnType=Mass  Density=1  DensityUnits=kg/m^3  DoExposeReferenceFrame=on  SerializedFrames=<Frames><Frame><Id>Frame1</Id><Value><Name>RL3_4</Name><Origin><Source>GeometricFeature</Source><FeatureName>planar surface 16</FeatureName></Origin><PrimaryAxis><DefinedDirection>+Z</DefinedDirection><Source>ReferenceFrame</Source><SourceDirection>+X</SourceDirection><FeatureName></FeatureName></PrimaryAxis><SecondaryAxis><DefinedDirection>+X</DefinedDirection><Source>ReferenceFrame</Source><SourceDirection>+Y</SourceDirection><FeatureName></FeatureName></SecondaryAxis></Value></Frame><Frame><Id>Frame2</Id><Value><Name>RL2</Name><Origin><Source>GeometricFeature</Source><FeatureName>circular curve 32</FeatureName></Origin><PrimaryAxis><DefinedDirection>+Z</DefinedDirection><Source>ReferenceFrame</Source><SourceDirection>-Z</SourceDirection><FeatureName></FeatureName></PrimaryAxis><SecondaryAxis><DefinedDirection>+X</DefinedDirection><Source>ReferenceFrame</Source><SourceDirection>+X</SourceDirection><FeatureName></FeatureName></SecondaryAxis></Value></Frame></Frames>  GraphicType=FromGeometry  MarkerShape=Sphere  MarkerSize=10  GraphicVisPropType=SimpleVisualProperties  GraphicDiffuseColor=[0.5 0.5 0.5]  GraphicSpecularColor=[0.5 0.5 0.5 1.0]  GraphicAmbientColor=[0.15 0.15 0.15 1.0]  GraphicEmissiveColor=[0.0 0.0 0.0 1.0]  GraphicShininess=75  GraphicOpacity=1.0
  riferimento_link3_2 : PMIOPort  Side=Left
  riferimento_link4_3 : PMIOPort  Port=2  Side=Right
  connections:
  riferimento_link3_2/RConn1 -- Rigid Transform/LConn1
  riferimento_link4_3/RConn1 -- Solid_link3/LConn1
  Solid_link3/LConn2 -- Rigid Transform/RConn1

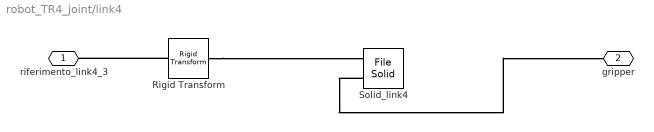
== system robot_TR4_joint/link4 ==
  Rigid Transform : sm_lib/Frames and Transforms/Rigid Transform  TranslationMethod=None  TranslationStandardOffset=0  TranslationLengthUnit=m  TranslationStandardAxis=+Z  TranslationCartesianOffset=[0 0 0]  TranslationROffset=0  TranslationROffsetUnits=m  TranslationZOffset=0  TranslationZOffsetUnits=m  TranslationThetaOffset=0  TranslationThetaOffsetUnits=deg  RotationMethod=StandardAxis  RotationAngleUnits=deg  RotationStandardAxis=+Z  RotationAngle=135  RotationArbitraryAxis=[0 0 1]  FollAlignAxisA=+X  BaseAlignAxisA=+Y  FollAlignAxisB=+Y  BaseAlignAxisB=+Z  RotationSequenceAxes=FollowerAxes  RotationSequence=XYX  RotationSequenceAngles=[0 0 0]  RotationSequenceAnglesUnits=deg  RotationMatrix=[1 0 0; 0 1 0; 0 0 1]
  Solid_link4 : sm_lib/Body Elements/File Solid  ExtGeomFileName=D:\repository\Servo_System_progetto\Solidworks\step\TR4link4.STEP  UnitType=FromFile  ExtGeomFileUnits=m  StepReaderType=HEX  ExportConvexHullGeometry=off  InertiaType=CalculateFromGeometry  Mass=3.19  MassUnits=g  CenterOfMass=[0 0 0]  CenterOfMassUnits=m  MomentsOfInertia=[1 1 1]  MomentsOfInertiaUnits=kg*m^2  ProductsOfInertia=[0 0 0]  ProductsOfInertiaUnits=kg*m^2  BasedOnType=Mass  Density=1  DensityUnits=kg/m^3  DoExposeReferenceFrame=on  SerializedFrames=<Frames><Frame><Id>Frame1</Id><Value><Name>link4</Name><Origin><Source>GeometricFeature</Source><FeatureName>circular curve 10</FeatureName></Origin><PrimaryAxis><DefinedDirection>+Z</DefinedDirection><Source>ReferenceFrame</Source><SourceDirection>+Y</SourceDirection><FeatureName></FeatureName></PrimaryAxis><SecondaryAxis><DefinedDirection>+X</DefinedDirection><Source>ReferenceFrame</Source><SourceDirection>+X</SourceDirection><FeatureName></FeatureName></SecondaryAxis></Value></Frame><Frame><Id>Frame2</Id><Value><Name>gripper</Name><Origin><Source>GeometricFeature</Source><FeatureName>planar surface 1</FeatureName></Origin><PrimaryAxis><DefinedDirection>+Z</DefinedDirection><Source>ReferenceFrame</Source><SourceDirection>+X</SourceDirection><FeatureName></FeatureName></PrimaryAxis><SecondaryAxis><DefinedDirection>+X</DefinedDirection><Source>ReferenceFrame</Source><SourceDirection>+Y</SourceDirection><FeatureName></FeatureName></SecondaryAxis></Value></Frame></Frames>  GraphicType=FromGeometry  MarkerShape=Sphere  MarkerSize=10  GraphicVisPropType=SimpleVisualProperties  GraphicDiffuseColor=[0.5 0.5 0.5]  GraphicSpecularColor=[0.5 0.5 0.5 1.0]  GraphicAmbientColor=[0.15 0.15 0.15 1.0]  GraphicEmissiveColor=[0.0 0.0 0.0 1.0]  GraphicShininess=75  GraphicOpacity=1.0
  riferimento_link4_3 : PMIOPort  Side=Left
  gripper : PMIOPort  Port=2  Side=Right
  connections:
  Solid_link4/LConn2 -- gripper/RConn1
  Rigid Transform/LConn1 -- riferimento_link4_3/RConn1
  Rigid Transform/RConn1 -- Solid_link4/LConn1

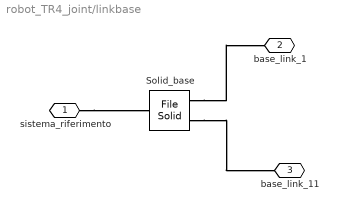
== system robot_TR4_joint/linkbase ==
  Solid_base : sm_lib/Body Elements/File Solid  ExtGeomFileName=D:\repository\Servo_System_progetto\Solidworks\step\TR4basemat.STEP  UnitType=FromFile  ExtGeomFileUnits=m  StepReaderType=HEX  ExportConvexHullGeometry=off  InertiaType=CalculateFromGeometry  Mass=126.25  MassUnits=g  CenterOfMass=[0 0 0]  CenterOfMassUnits=m  MomentsOfInertia=[1 1 1]  MomentsOfInertiaUnits=kg*m^2  ProductsOfInertia=[0 0 0]  ProductsOfInertiaUnits=kg*m^2  BasedOnType=Mass  Density=1  DensityUnits=kg/m^3  DoExposeReferenceFrame=on  SerializedFrames=<Frames><Frame><Id>Frame1</Id><Value><Name>RB1</Name><Origin><Source>GeometricFeature</Source><FeatureName>circular curve 8</FeatureName></Origin><PrimaryAxis><DefinedDirection>+Z</DefinedDirection><Source>ReferenceFrame</Source><SourceDirection>-Z</SourceDirection><FeatureName></FeatureName></PrimaryAxis><SecondaryAxis><DefinedDirection>+X</DefinedDirection><Source>ReferenceFrame</Source><SourceDirection>+X</SourceDirection><FeatureName></FeatureName></SecondaryAxis></Value></Frame><Frame><Id>Frame2</Id><Value><Name>RB2</Name><Origin><Source>GeometricFeature</Source><FeatureName>circular curve 6</FeatureName></Origin><PrimaryAxis><DefinedDirection>-Z</DefinedDirection><Source>GeometricFeature</Source><SourceDirection>+Z</SourceDirection><FeatureName>segment 6</FeatureName></PrimaryAxis><SecondaryAxis><DefinedDirection>+X</DefinedDirection><Source>ReferenceFrame</Source><SourceDirection>+X</SourceDirection><FeatureName></FeatureName></SecondaryAxis></Value></Frame></Frames>  GraphicType=FromGeometry  MarkerShape=Sphere  MarkerSize=10  GraphicVisPropType=SimpleVisualProperties  GraphicDiffuseColor=[0.5 0.5 0.5]  GraphicSpecularColor=[0.5 0.5 0.5 1.0]  GraphicAmbientColor=[0.15 0.15 0.15 1.0]  GraphicEmissiveColor=[0.0 0.0 0.0 1.0]  GraphicShininess=75  GraphicOpacity=1.0
  sistema_riferimento : PMIOPort  Side=Left
  base_link_1 : PMIOPort  Port=2  Side=Right
  base_link_11 : PMIOPort  Port=3  Side=Right
  connections:
  sistema_riferimento/RConn1 -- Solid_base/RConn1
  Solid_base/LConn1 -- base_link_1/RConn1
  Solid_base/LConn2 -- base_link_11/RConn1

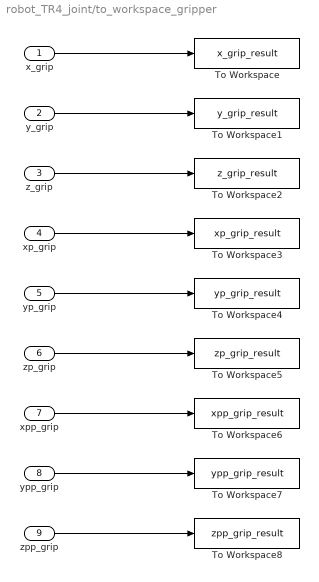
== system robot_TR4_joint/to_workspace_gripper ==
  x_grip : Inport
  y_grip : Inport  Port=2
  z_grip : Inport  Port=3
  xp_grip : Inport  Port=4
  yp_grip : Inport  Port=5
  zp_grip : Inport  Port=6
  xpp_grip : Inport  Port=7
  ypp_grip : Inport  Port=8
  zpp_grip : Inport  Port=9
  To Workspace : ToWorkspace  VariableName=x_grip_result  SaveFormat=Timeseries  SampleTime=-1
  To Workspace1 : ToWorkspace  VariableName=y_grip_result  SaveFormat=Timeseries  SampleTime=-1
  To Workspace2 : ToWorkspace  VariableName=z_grip_result  SaveFormat=Timeseries  SampleTime=-1
  To Workspace3 : ToWorkspace  VariableName=xp_grip_result  SaveFormat=Timeseries  SampleTime=-1
  To Workspace4 : ToWorkspace  VariableName=yp_grip_result  SaveFormat=Timeseries  SampleTime=-1
  To Workspace5 : ToWorkspace  VariableName=zp_grip_result  SaveFormat=Timeseries  SampleTime=-1
  To Workspace6 : ToWorkspace  VariableName=xpp_grip_result  SaveFormat=Timeseries  SampleTime=-1
  To Workspace7 : ToWorkspace  VariableName=ypp_grip_result  SaveFormat=Timeseries  SampleTime=-1
  To Workspace8 : ToWorkspace  VariableName=zpp_grip_result  SaveFormat=Timeseries  SampleTime=-1
  wires:
  x_grip/1 -> To Workspace/1
  y_grip/1 -> To Workspace1/1
  z_grip/1 -> To Workspace2/1
  xp_grip/1 -> To Workspace3/1
  zp_grip/1 -> To Workspace5/1
  yp_grip/1 -> To Workspace4/1
  xpp_grip/1 -> To Workspace6/1
  zpp_grip/1 -> To Workspace8/1
  ypp_grip/1 -> To Workspace7/1

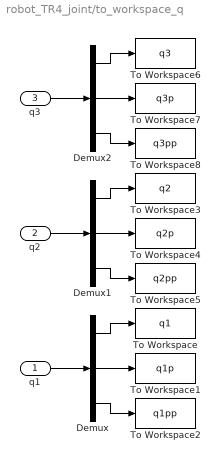
== system robot_TR4_joint/to_workspace_q ==
  q1 : Inport
  q2 : Inport  Port=2
  q3 : Inport  Port=3
  Demux : Demux  Outputs=3
  Demux1 : Demux  Outputs=3
  Demux2 : Demux  Outputs=3
  To Workspace : ToWorkspace  VariableName=q1  SaveFormat=Timeseries  SampleTime=-1
  To Workspace1 : ToWorkspace  VariableName=q1p  SaveFormat=Timeseries  SampleTime=-1
  To Workspace2 : ToWorkspace  VariableName=q1pp  SaveFormat=Timeseries  SampleTime=-1
  To Workspace3 : ToWorkspace  VariableName=q2  SaveFormat=Timeseries  SampleTime=-1
  To Workspace4 : ToWorkspace  VariableName=q2p  SaveFormat=Timeseries  SampleTime=-1
  To Workspace5 : ToWorkspace  VariableName=q2pp  SaveFormat=Timeseries  SampleTime=-1
  To Workspace6 : ToWorkspace  VariableName=q3  SaveFormat=Timeseries  SampleTime=-1
  To Workspace7 : ToWorkspace  VariableName=q3p  SaveFormat=Timeseries  SampleTime=-1
  To Workspace8 : ToWorkspace  VariableName=q3pp  SaveFormat=Timeseries  SampleTime=-1
  wires:
  Demux/1 -> To Workspace/1
  Demux1/1 -> To Workspace3/1
  Demux/2 -> To Workspace1/1
  Demux1/2 -> To Workspace4/1
  Demux/3 -> To Workspace2/1
  Demux1/3 -> To Workspace5/1
  q1/1 -> Demux/1
  q2/1 -> Demux1/1
  q3/1 -> Demux2/1
  Demux2/1 -> To Workspace6/1
  Demux2/2 -> To Workspace7/1
  Demux2/3 -> To Workspace8/1

== matlab function robot_TR4_joint/Trajectory Generator ==
  data: t input; dT_target parameter; q1 output; q1p output; q1pp output; q2 output; q2p output; q2pp output; q3 output; q3p output; q3pp output; Q_interp parameter; Qp_interp parameter; Qpp_interp parameter; Fq1 output; Fq2 output; Fq3 output; Fq_interp parameter
function [q1, q1p,q1pp,q2,q2p,q2pp,q3,q3p,q3pp,Fq1,Fq2,Fq3] = traj_gen(t,dT_target, ...
                                    Q_interp,Qp_interp,Qpp_interp,Fq_interp)

                                
    val=find(dT_target<=t);
    indice=val(end);                         
    
    q1 = Q_interp(indice,1);
    q2 = Q_interp(indice,2);
    q3 = Q_interp(indice,3);
    q1p = Qp_interp(indice,1);
    q2p = Qp_interp(indice,2);
    q3p = Qp_interp(indice,3);
    q1pp = Qpp_interp(indice,1);
    q2pp = Qpp_interp(indice,2);
    q3pp = Qpp_interp(indice,3);
  
    Fq1 = 0;
    Fq2 = 0;
    Fq3 = 0;
end
